simulink library "csc_gal_gdn_approach_landing_lib"  (R2015b)
settings: Solver=ode45  StartTime=0.0  StopTime=10.0  RelTol=1e-3
values from neighbouring files (symbols this model uses):
  ltg_minimum_pulse_width_milliseconds = 60    [csc_ltg_landing_terminal_guidance_init.m]
undefined symbols (not defined in the file or in its folder): gdn_millisec_per_cycle
libraries: util_common_lib x4, util_quat_lib x4, util_info_lib x1, csc_lac_landing_acceleration_command_lib x1, csu_arg_aimpoint_roll_guidance_lib x1
settings Model: Creator=Nilesh  LastModifiedBy=jkaidy
settings DataIOCC: SaveFormat=Array
settings DebuggingCC: UnderspecifiedInitializationDetection=Classic  MergeDetectMultiDrivingBlocksExec=none  SolverPrmCheckMsg=warning  StateNameClashWarn=warning
settings HardwareCC: ProdBitPerPointer=32  ProdLargestAtomicFloat=None  ProdIntDivRoundTo=Undefined  ProdEndianess=Unspecified  ProdWordSize=32  ProdHWDeviceType=32-bit Generic
settings GRTTargetCC: GeneratePreprocessorConditionals=Disable all
settings ConfigComp: CovModelRefEnable=Off  CovSFcnEnable=off

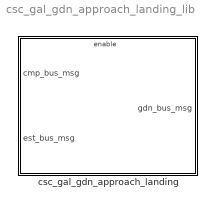
== system csc_gal_gdn_approach_landing_lib ==
  csc_gal_gdn_approach_landing : Subsystem

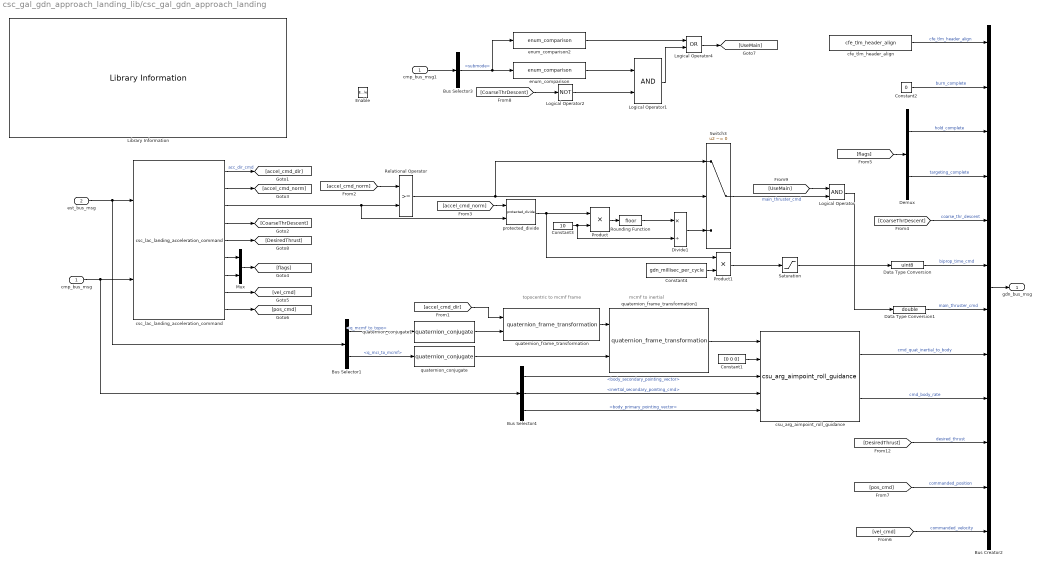
== system csc_gal_gdn_approach_landing_lib/csc_gal_gdn_approach_landing ==
  note: mcmf to inertial
  note: topocentric to mcmf frame
  cmp_bus_msg : Inport
  est_bus_msg : Inport  Port=2
  Enable : EnablePort
  Bus Selector1 : BusSelector  OutputSignals=q_mcmf_to_topo,q_mci_to_mcmf
  Bus Selector3 : BusSelector  OutputSignals=submode
  Bus Selector4 : BusSelector  OutputSignals=body_secondary_pointing_vector,inertial_secondary_pointing_cmd,body_primary_pointing_vector
  Bus Creator2 : BusCreator  Inputs=12  OutDataTypeStr=Bus: gdn_bus_msg  NonVirtualBus=on
  Constant1 : Constant  Value=[0 0 0]  SampleTime=-1
  Constant2 : Constant  Value=0  OutDataTypeStr=uint8
  Constant3 : Constant  Value=10
  Constant4 : Constant  Value=gdn_millisec_per_cycle
  Data Type Conversion : DataTypeConversion  OutDataTypeStr=uint8
  Data Type Conversion1 : DataTypeConversion  OutDataTypeStr=double
  Demux : Demux  Outputs=2
  Divide1 : Product  Inputs=*/
  Library Information : util_info_lib/Library Information  owner='NONE'
  Logical Operator : Logic  AllPortsSameDT=off  OutDataTypeStr=boolean
  Logical Operator1 : Logic  AllPortsSameDT=off  OutDataTypeStr=boolean
  Logical Operator2 : Logic  Operator=NOT  AllPortsSameDT=off  OutDataTypeStr=boolean
  Logical Operator4 : Logic  Operator=OR  AllPortsSameDT=off  OutDataTypeStr=boolean
  Mux : Mux  Inputs=2
  Product : Product  RndMeth=Zero
  Product1 : Product
  Relational Operator : RelationalOperator  OutDataTypeStr=boolean
  Rounding Function : Rounding
  Saturation : Saturate  UpperLimit=gdn_millisec_per_cycle  LowerLimit=ltg_minimum_pulse_width_milliseconds
  Switch3 : Switch  Criteria=u2 ~= 0
  cfe_tlm_header_align : util_common_lib/cfe_tlm_header_align
  cmp_bus_msg1 : InportShadow
  csc_lac_landing_acceleration_command : csc_lac_landing_acceleration_command_lib/csc_lac_landing_acceleration_command
  csu_arg_aimpoint_roll_guidance : csu_arg_aimpoint_roll_guidance_lib/csu_arg_aimpoint_roll_guidance
  enum_comparison : util_common_lib/enum_comparison  comparison_type===
  enum_comparison2 : util_common_lib/enum_comparison  comparison_type===
  protected_divide : util_common_lib/protected_divide  fault_value=0  tolerance=eps
  quaternion_conjugate : util_quat_lib/quaternion_conjugate  SystemSampleTime=-1
  quaternion_conjugate1 : util_quat_lib/quaternion_conjugate  SystemSampleTime=-1
  quaternion_frame_transformation : util_quat_lib/quaternion_frame_transformation  SystemSampleTime=-1
  quaternion_frame_transformation1 : util_quat_lib/quaternion_frame_transformation  SystemSampleTime=-1
  gdn_bus_msg : Outport  OutDataTypeStr=Bus: gdn_bus_msg  OutputWhenDisabled=reset  InitialOutput=0
  wires:
  Constant2/1 -> Bus Creator2/2  "burn_complete"
  Logical Operator/1 -> Data Type Conversion1/1
  Product1/1 -> Saturation/1
  [DesiredThrust] -> Bus Creator2/10  "desired_thrust"
  [pos_cmd] -> Bus Creator2/11  "commanded_position"
  [vel_cmd] -> Bus Creator2/12  "commanded_velocity"
  csc_lac_landing_acceleration_command/9 -> [pos_cmd]
  csc_lac_landing_acceleration_command/8 -> [vel_cmd]
  Data Type Conversion/1 -> Bus Creator2/6  "biprop_time_cmd"
  cfe_tlm_header_align/1 -> Bus Creator2/1  "cfe_tlm_header_align"
  csc_lac_landing_acceleration_command/7 -> Mux/2
  csc_lac_landing_acceleration_command/6 -> Mux/1
  Demux/1 -> Bus Creator2/3  "hold_complete"
  Demux/2 -> Bus Creator2/4  "targeting_complete"
  [flags] -> Demux/1
  Mux/1 -> [flags]
  [accel_cmd_norm] -> protected_divide/1
  [accel_cmd_norm] -> Relational Operator/1
  csc_lac_landing_acceleration_command/2 -> [accel_cmd_norm]
  [accel_cmd_dir] -> quaternion_frame_transformation/1
  Bus Selector1/2 -> quaternion_conjugate/1  "<q_mci_to_mcmf>"
  Bus Selector1/1 -> quaternion_conjugate1/1  "<q_mcmf_to_topo>"
  Bus Selector4/1 -> csu_arg_aimpoint_roll_guidance/3  "<body_secondary_pointing_vector>"
  csu_arg_aimpoint_roll_guidance/2 -> Bus Creator2/9  "cmd_body_rate"
  csu_arg_aimpoint_roll_guidance/1 -> Bus Creator2/8  "cmd_quat_inertial_to_body"
  quaternion_frame_transformation1/1 -> csu_arg_aimpoint_roll_guidance/1
  Bus Creator2/1 -> gdn_bus_msg/1
  quaternion_conjugate/1 -> quaternion_frame_transformation1/2
  quaternion_conjugate1/1 -> quaternion_frame_transformation/2
  quaternion_frame_transformation/1 -> quaternion_frame_transformation1/1
  csc_lac_landing_acceleration_command/3 -> Relational Operator/2, protected_divide/2
  Constant3/1 -> Product/2, Divide1/2
  Product/1 -> Rounding Function/1
  Rounding Function/1 -> Divide1/1
  Divide1/1 -> Switch3/3
  cmp_bus_msg/1 -> csc_lac_landing_acceleration_command/2, Bus Selector4/1
  est_bus_msg/1 -> csc_lac_landing_acceleration_command/1, Bus Selector1/1
  Constant1/1 -> csu_arg_aimpoint_roll_guidance/2
  Bus Selector4/3 -> csu_arg_aimpoint_roll_guidance/5  "<body_primary_pointing_vector>"
  [CoarseThrDescent] -> Bus Creator2/5  "coarse_thr_descent"
  csc_lac_landing_acceleration_command/5 -> [DesiredThrust]
  Bus Selector4/2 -> csu_arg_aimpoint_roll_guidance/4  "<inertial_secondary_pointing_cmd>"
  csc_lac_landing_acceleration_command/1 -> [accel_cmd_dir]  "acc_dir_cmd"
  protected_divide/1 -> Product1/1, Product/1
  Constant4/1 -> Product1/2
  Saturation/1 -> Data Type Conversion/1
  cmp_bus_msg1/1 -> Bus Selector3/1
  Bus Selector3/1 -> enum_comparison2/1, enum_comparison/1  "<submode>"
  Relational Operator/1 -> Switch3/1, Switch3/2
  Switch3/1 -> Logical Operator/2  "main_thruster_cmd"
  [UseMain] -> Logical Operator/1
  Data Type Conversion1/1 -> Bus Creator2/7  "main_thruster_cmd"
  csc_lac_landing_acceleration_command/4 -> [CoarseThrDescent]
  [CoarseThrDescent] -> Logical Operator2/1
  Logical Operator2/1 -> Logical Operator1/2
  Logical Operator4/1 -> [UseMain]
  enum_comparison/1 -> Logical Operator1/1
  Logical Operator1/1 -> Logical Operator4/2
  enum_comparison2/1 -> Logical Operator4/1
